simulink model "Modbus_Fixed_Breaker"  (Simulink 8.1)
settings: Solver=ode45  StartTime=0.0  StopTime=10.0  RelTol=1e-3
undefined symbols (not defined in the file or in its folder): Ts
libraries: powerlib x16, powerlib_extras x16, dspsigops x4, breakers_1ph_3ph x4, rtio_generic_modbus x4
settings Model: Creator=AI24004  LastModifiedBy=ed12083
settings DebuggingCC: FcnCallInpInsideContextMsg=EnableAllAsWarning

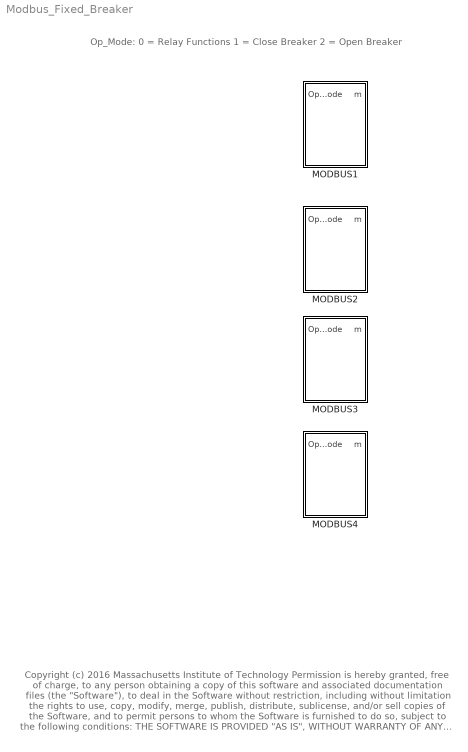
== system Modbus_Fixed_Breaker ==
  note: Op_Mode:
      | 0 = Relay Functions
      | 1 = Close Breaker
      | 2 = Open Breaker
  note: Copyright (c) 2016 Massachusetts Institute of Technology
      | Permission is hereby granted, free of charge, to any person obtaining a copy of this software and associated documentation files (the "Software"), to deal
      | in the Software without restriction, including without limitation the rights to use, copy, modify, merge, publish, distribute, sublicense, and/or sell copies of the
      | Software, and to permit persons to whom the Software is furnished to do so, subject to the following conditions:
      |
      | THE SOFTWARE IS PROVIDED "AS IS", WITHOUT WARRANTY OF ANY KIND, EXPRESS OR IMPLIED, INCLUDING BUT NOT LIMITED TO THE
      | WARRANTIES OF MERCHANTABILITY, FITNESS FOR A PARTICULAR PURPOSE AND NONINFRINGEMENT. IN NO EVENT SHALL THE AUTHORS
      | OR COPYRIGHT HOLDERS BE LIABLE FOR ANY CLAIM, DAMAGES OR OTHER LIABILITY, WHETHER IN AN ACTION OF CONTRACT, TORT OR
      | OTHERWISE, ARISING FROM, OUT OF OR IN CONNECTION WITH THE SOFTWARE OR THE USE OR OTHER DEALINGS IN THE SOFTWARE
  MODBUS1 : Subsystem  AncestorBlock=breakers_1ph_3ph/Protection  mask(Protection and Metering){IOC=15E3, TOC=1800, Ts=Ts, VRMSLL=13800, I_nom=200}
      mask prompts: IOC "IOC setting [A]"; TOC "TOC setting [A]"; Ts "Sampling Time [Sec]"; VRMSLL "Nominal Voltage [VRMSLL]"; I_nom "Continous Current [A]"
      mask help:
      | This block simulates the behavior of selected relay functions as well as metering equipment.
      | The block is intended to communicate with a microgrid controller providing it measurements, and switching controls.
      |
      | Supported relay functions (as of 06-15-2015):
      | 50/51: instantaneous and time-inverse overcurrent protection (moderate curve)
      mask Help:
      | This block simulates the behavior of selected relay functions as well as metering equipment (60 Hz - only).
      | The block is intended to communicate with a microgrid controller providing it measurements, and switching controls.
      | 
      | Supported relay functions (as of 06-15-2015):
      | 50/51: instantaneous and time-inverse overcurrent protection (moderate curve)
      | 
      | The input parameters are:
      | 0) Ts:  Sampling time [Seconds]
      | 1) State: 0 for relay logic mode, 1 to close the controlled breaker/switch,
      | and 2 to open the controlled breaker/switch
      | 2) TOC: Time-inverse overcurrent setting [Amperes]
      | 3) IOC: Instantaneous overcurrent setting [Amperes]
      | 
      | Metered parameters are:
      | 0) Status (0-closed, 1-open)
      | 1) Instantaneous voltage (abc)
      | 2) Instantaneous current (abc)
  MODBUS2 : Subsystem  AncestorBlock=breakers_1ph_3ph/Protection  mask(Protection and Metering){IOC=15E3, TOC=1800, Ts=Ts, VRMSLL=13800, I_nom=200}
      mask prompts: IOC "IOC setting [A]"; TOC "TOC setting [A]"; Ts "Sampling Time [Sec]"; VRMSLL "Nominal Voltage [VRMSLL]"; I_nom "Continous Current [A]"
      mask help:
      | This block simulates the behavior of selected relay functions as well as metering equipment.
      | The block is intended to communicate with a microgrid controller providing it measurements, and switching controls.
      |
      | Supported relay functions (as of 06-15-2015):
      | 50/51: instantaneous and time-inverse overcurrent protection (moderate curve)
      mask Help:
      | This block simulates the behavior of selected relay functions as well as metering equipment (60 Hz - only).
      | The block is intended to communicate with a microgrid controller providing it measurements, and switching controls.
      | 
      | Supported relay functions (as of 06-15-2015):
      | 50/51: instantaneous and time-inverse overcurrent protection (moderate curve)
      | 
      | The input parameters are:
      | 0) Ts:  Sampling time [Seconds]
      | 1) State: 0 for relay logic mode, 1 to close the controlled breaker/switch,
      | and 2 to open the controlled breaker/switch
      | 2) TOC: Time-inverse overcurrent setting [Amperes]
      | 3) IOC: Instantaneous overcurrent setting [Amperes]
      | 
      | Metered parameters are:
      | 0) Status (0-closed, 1-open)
      | 1) Instantaneous voltage (abc)
      | 2) Instantaneous current (abc)
  MODBUS3 : Subsystem  AncestorBlock=breakers_1ph_3ph/Protection  mask(Protection and Metering){IOC=15E3, TOC=1800, Ts=Ts, VRMSLL=13800, I_nom=200}
      mask prompts: IOC "IOC setting [A]"; TOC "TOC setting [A]"; Ts "Sampling Time [Sec]"; VRMSLL "Nominal Voltage [VRMSLL]"; I_nom "Continous Current [A]"
      mask help:
      | This block simulates the behavior of selected relay functions as well as metering equipment.
      | The block is intended to communicate with a microgrid controller providing it measurements, and switching controls.
      |
      | Supported relay functions (as of 06-15-2015):
      | 50/51: instantaneous and time-inverse overcurrent protection (moderate curve)
      mask Help:
      | This block simulates the behavior of selected relay functions as well as metering equipment (60 Hz - only).
      | The block is intended to communicate with a microgrid controller providing it measurements, and switching controls.
      | 
      | Supported relay functions (as of 06-15-2015):
      | 50/51: instantaneous and time-inverse overcurrent protection (moderate curve)
      | 
      | The input parameters are:
      | 0) Ts:  Sampling time [Seconds]
      | 1) State: 0 for relay logic mode, 1 to close the controlled breaker/switch,
      | and 2 to open the controlled breaker/switch
      | 2) TOC: Time-inverse overcurrent setting [Amperes]
      | 3) IOC: Instantaneous overcurrent setting [Amperes]
      | 
      | Metered parameters are:
      | 0) Status (0-closed, 1-open)
      | 1) Instantaneous voltage (abc)
      | 2) Instantaneous current (abc)
  MODBUS4 : Subsystem  AncestorBlock=breakers_1ph_3ph/Protection  mask(Protection and Metering){IOC=15E3, TOC=1800, Ts=Ts, VRMSLL=13800, I_nom=200}
      mask prompts: IOC "IOC setting [A]"; TOC "TOC setting [A]"; Ts "Sampling Time [Sec]"; VRMSLL "Nominal Voltage [VRMSLL]"; I_nom "Continous Current [A]"
      mask help:
      | This block simulates the behavior of selected relay functions as well as metering equipment.
      | The block is intended to communicate with a microgrid controller providing it measurements, and switching controls.
      |
      | Supported relay functions (as of 06-15-2015):
      | 50/51: instantaneous and time-inverse overcurrent protection (moderate curve)
      mask Help:
      | This block simulates the behavior of selected relay functions as well as metering equipment (60 Hz - only).
      | The block is intended to communicate with a microgrid controller providing it measurements, and switching controls.
      | 
      | Supported relay functions (as of 06-15-2015):
      | 50/51: instantaneous and time-inverse overcurrent protection (moderate curve)
      | 
      | The input parameters are:
      | 0) Ts:  Sampling time [Seconds]
      | 1) State: 0 for relay logic mode, 1 to close the controlled breaker/switch,
      | and 2 to open the controlled breaker/switch
      | 2) TOC: Time-inverse overcurrent setting [Amperes]
      | 3) IOC: Instantaneous overcurrent setting [Amperes]
      | 
      | Metered parameters are:
      | 0) Status (0-closed, 1-open)
      | 1) Instantaneous voltage (abc)
      | 2) Instantaneous current (abc)

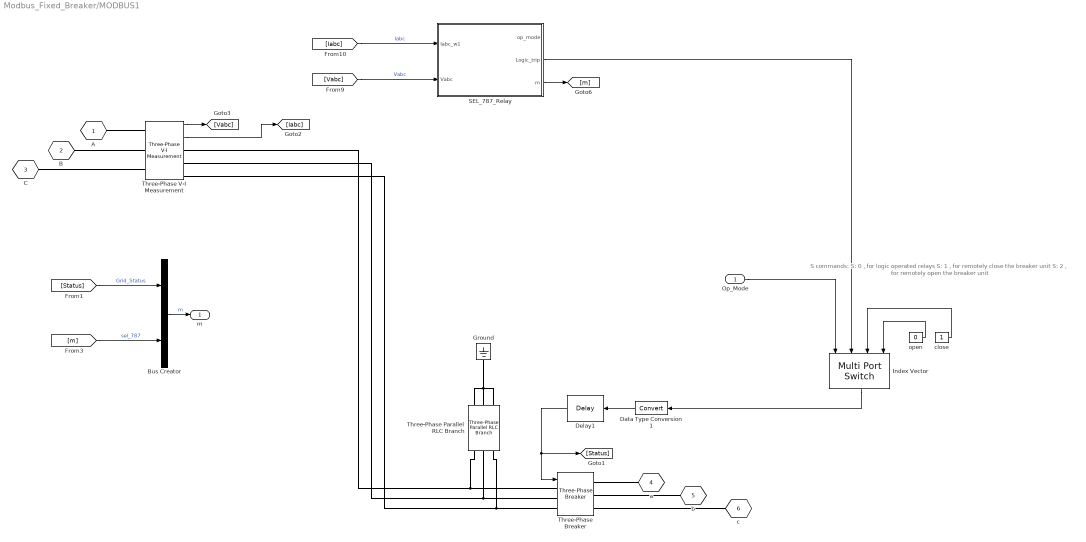
== system Modbus_Fixed_Breaker/MODBUS1 ==
  note: S commands:
      | S: 0 , for logic operated relays
      | S: 1 ,  for remotely close the breaker unit
      | S: 2 , for remotely open the breaker unit
  Op_Mode : Inport
  Bus Creator : BusCreator  Inputs=2
  Data Type Conversion1 : DataTypeConversion
  Delay1 : dspsigops/Delay  dly_unit=Samples  delay=lower((3/60)/Ts)  ic_detail=off  dif_ic_for_ch=off  dif_ic_for_dly=off  ic=1  reset_popup=None
  Ground : powerlib/Elements/Ground  LConnTagsString=a
  Index Vector : MultiPortSwitch  DataPortOrder=Zero-based contiguous  DataPortIndices={2,1,0}  zeroidx=on
  SEL_787_Relay : Subsystem
  Three-Phase Parallel RLC Branch : powerlib/Elements/Three-Phase Parallel RLC Branch  LConnTagsString=A|B|C  RConnTagsString=A|B|C  BranchType=RLC  Resistance=10e6  Inductance=1e-3  Capacitance=1e-6  Measurements=None
  Three-Phase V-I Measurement : powerlib/Measurements/Three-Phase V-I Measurement  VoltageMeasurement=phase-to-ground  SetLabelV=off  LabelV=Vabc  Vpu=off  VpuLL=off  CurrentMeasurement=yes  SetLabelI=off  LabelI=Iabc  Ipu=off  Pbase=100e6  Vbase=500e3  OutputType=Complex  PhasorSimulation=off  PSBequivalent=0
  Three-Phase Breaker : powerlib/Elements/Three-Phase Breaker  InitialState=closed  SwitchA=on  SwitchB=on  SwitchC=on  SwitchTimes="[1/60  5/60]"  External=on  BreakerResistance=1e-3  SnubberResistance=1e8  SnubberCapacitance=inf  Measurements=None
  close : Constant
  open : Constant  Value=0
  A : PMIOPort  Tag=PMCPort  Port=1  Side=Left
  B : PMIOPort  Tag=PMCPort  Port=2  Side=Left
  C : PMIOPort  Tag=PMCPort  Port=3  Side=Left
  a : PMIOPort  Tag=PMCPort  Port=4  Side=Right
  b : PMIOPort  Tag=PMCPort  Port=5  Side=Right
  c : PMIOPort  Tag=PMCPort  Port=6  Side=Right
  m : Outport
  wires:
  [m] -> Bus Creator/2  "sel_787"
  SEL_787_Relay/3(m) -> [m]
  Bus Creator/1 -> m/1  "m"
  [Status] -> Bus Creator/1  "Grid_Status"
  Delay1/1 -> [Status], Three-Phase Breaker/1
  Three-Phase V-I Measurement/1 -> [Vabc]
  Three-Phase V-I Measurement/2 -> [Iabc]
  open/1 -> Index Vector/4
  close/1 -> Index Vector/3
  Index Vector/1 -> Data Type Conversion1/1
  Data Type Conversion1/1 -> Delay1/1
  [Iabc] -> SEL_787_Relay/1(Iabc_w1)  "Iabc"
  [Vabc] -> SEL_787_Relay/2(Vabc)  "Vabc"
  SEL_787_Relay/2(Logic_trip) -> Index Vector/2
  Op_Mode/1 -> Index Vector/1
  connections:
  Three-Phase Parallel RLC Branch/RConn1 -- Three-Phase Breaker/LConn1 -- Three-Phase V-I Measurement/RConn1
  Three-Phase Parallel RLC Branch/RConn2 -- Three-Phase Breaker/LConn2 -- Three-Phase V-I Measurement/RConn2
  Three-Phase Parallel RLC Branch/RConn3 -- Three-Phase Breaker/LConn3 -- Three-Phase V-I Measurement/RConn3
  Three-Phase Breaker/RConn2 -- b/RConn1
  Three-Phase Breaker/RConn3 -- c/RConn1
  Three-Phase V-I Measurement/LConn1 -- A/RConn1
  a/RConn1 -- Three-Phase Breaker/RConn1
  C/RConn1 -- Three-Phase V-I Measurement/LConn3
  B/RConn1 -- Three-Phase V-I Measurement/LConn2
  Ground/LConn1 -- Three-Phase Parallel RLC Branch/LConn2 -- Three-Phase Parallel RLC Branch/LConn3 -- Three-Phase Parallel RLC Branch/LConn1

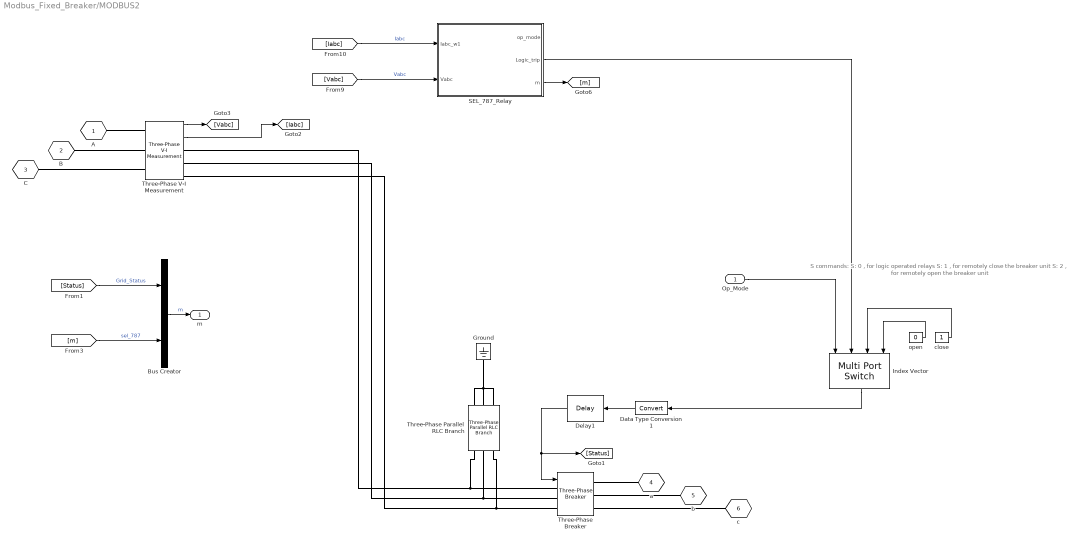
== system Modbus_Fixed_Breaker/MODBUS2 ==
  note: S commands:
      | S: 0 , for logic operated relays
      | S: 1 ,  for remotely close the breaker unit
      | S: 2 , for remotely open the breaker unit
  Op_Mode : Inport
  Bus Creator : BusCreator  Inputs=2
  Data Type Conversion1 : DataTypeConversion
  Delay1 : dspsigops/Delay  dly_unit=Samples  delay=lower((3/60)/Ts)  ic_detail=off  dif_ic_for_ch=off  dif_ic_for_dly=off  ic=1  reset_popup=None
  Ground : powerlib/Elements/Ground  LConnTagsString=a
  Index Vector : MultiPortSwitch  DataPortOrder=Zero-based contiguous  DataPortIndices={2,1,0}  zeroidx=on
  SEL_787_Relay : Subsystem
  Three-Phase Parallel RLC Branch : powerlib/Elements/Three-Phase Parallel RLC Branch  LConnTagsString=A|B|C  RConnTagsString=A|B|C  BranchType=RLC  Resistance=10e6  Inductance=1e-3  Capacitance=1e-6  Measurements=None
  Three-Phase V-I Measurement : powerlib/Measurements/Three-Phase V-I Measurement  VoltageMeasurement=phase-to-ground  SetLabelV=off  LabelV=Vabc  Vpu=off  VpuLL=off  CurrentMeasurement=yes  SetLabelI=off  LabelI=Iabc  Ipu=off  Pbase=100e6  Vbase=500e3  OutputType=Complex  PhasorSimulation=off  PSBequivalent=0
  Three-Phase Breaker : powerlib/Elements/Three-Phase Breaker  InitialState=closed  SwitchA=on  SwitchB=on  SwitchC=on  SwitchTimes="[1/60  5/60]"  External=on  BreakerResistance=1e-3  SnubberResistance=1e8  SnubberCapacitance=inf  Measurements=None
  close : Constant
  open : Constant  Value=0
  A : PMIOPort  Tag=PMCPort  Port=1  Side=Left
  B : PMIOPort  Tag=PMCPort  Port=2  Side=Left
  C : PMIOPort  Tag=PMCPort  Port=3  Side=Left
  a : PMIOPort  Tag=PMCPort  Port=4  Side=Right
  b : PMIOPort  Tag=PMCPort  Port=5  Side=Right
  c : PMIOPort  Tag=PMCPort  Port=6  Side=Right
  m : Outport
  wires:
  [m] -> Bus Creator/2  "sel_787"
  SEL_787_Relay/3(m) -> [m]
  Bus Creator/1 -> m/1  "m"
  [Status] -> Bus Creator/1  "Grid_Status"
  Delay1/1 -> [Status], Three-Phase Breaker/1
  Three-Phase V-I Measurement/1 -> [Vabc]
  Three-Phase V-I Measurement/2 -> [Iabc]
  open/1 -> Index Vector/4
  close/1 -> Index Vector/3
  Index Vector/1 -> Data Type Conversion1/1
  Data Type Conversion1/1 -> Delay1/1
  [Iabc] -> SEL_787_Relay/1(Iabc_w1)  "Iabc"
  [Vabc] -> SEL_787_Relay/2(Vabc)  "Vabc"
  SEL_787_Relay/2(Logic_trip) -> Index Vector/2
  Op_Mode/1 -> Index Vector/1
  connections:
  Three-Phase V-I Measurement/RConn1 -- Three-Phase Parallel RLC Branch/RConn1 -- Three-Phase Breaker/LConn1
  Three-Phase V-I Measurement/RConn2 -- Three-Phase Parallel RLC Branch/RConn2 -- Three-Phase Breaker/LConn2
  Three-Phase V-I Measurement/RConn3 -- Three-Phase Parallel RLC Branch/RConn3 -- Three-Phase Breaker/LConn3
  Three-Phase Breaker/RConn2 -- b/RConn1
  Three-Phase Breaker/RConn3 -- c/RConn1
  Three-Phase V-I Measurement/LConn1 -- A/RConn1
  a/RConn1 -- Three-Phase Breaker/RConn1
  C/RConn1 -- Three-Phase V-I Measurement/LConn3
  B/RConn1 -- Three-Phase V-I Measurement/LConn2
  Ground/LConn1 -- Three-Phase Parallel RLC Branch/LConn2 -- Three-Phase Parallel RLC Branch/LConn3 -- Three-Phase Parallel RLC Branch/LConn1

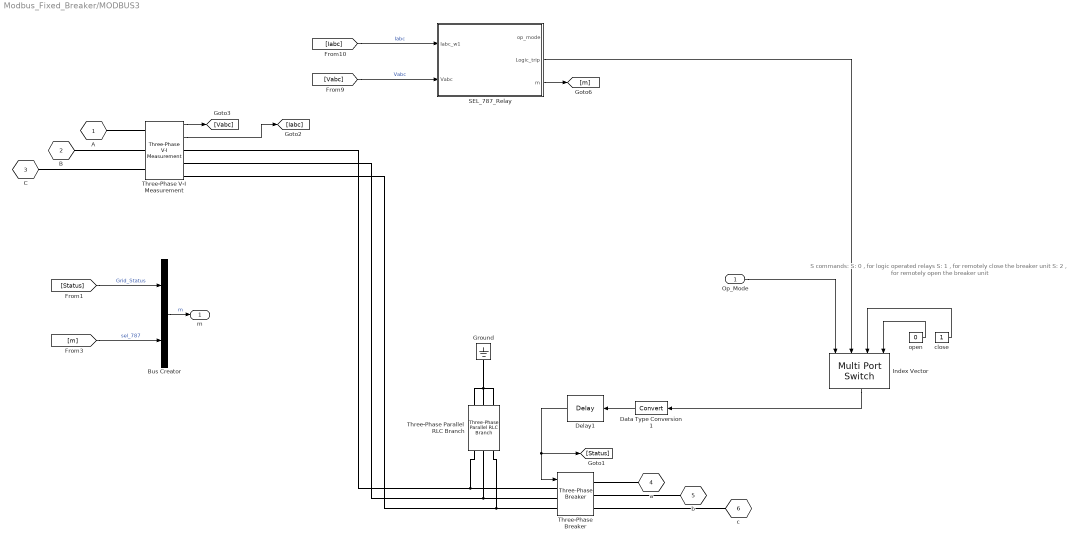
== system Modbus_Fixed_Breaker/MODBUS3 ==
  note: S commands:
      | S: 0 , for logic operated relays
      | S: 1 ,  for remotely close the breaker unit
      | S: 2 , for remotely open the breaker unit
  Op_Mode : Inport
  Bus Creator : BusCreator  Inputs=2
  Data Type Conversion1 : DataTypeConversion
  Delay1 : dspsigops/Delay  dly_unit=Samples  delay=lower((3/60)/Ts)  ic_detail=off  dif_ic_for_ch=off  dif_ic_for_dly=off  ic=1  reset_popup=None
  Ground : powerlib/Elements/Ground  LConnTagsString=a
  Index Vector : MultiPortSwitch  DataPortOrder=Zero-based contiguous  DataPortIndices={2,1,0}  zeroidx=on
  SEL_787_Relay : Subsystem
  Three-Phase Parallel RLC Branch : powerlib/Elements/Three-Phase Parallel RLC Branch  LConnTagsString=A|B|C  RConnTagsString=A|B|C  BranchType=RLC  Resistance=10e6  Inductance=1e-3  Capacitance=1e-6  Measurements=None
  Three-Phase V-I Measurement : powerlib/Measurements/Three-Phase V-I Measurement  VoltageMeasurement=phase-to-ground  SetLabelV=off  LabelV=Vabc  Vpu=off  VpuLL=off  CurrentMeasurement=yes  SetLabelI=off  LabelI=Iabc  Ipu=off  Pbase=100e6  Vbase=500e3  OutputType=Complex  PhasorSimulation=off  PSBequivalent=0
  Three-Phase Breaker : powerlib/Elements/Three-Phase Breaker  InitialState=closed  SwitchA=on  SwitchB=on  SwitchC=on  SwitchTimes="[1/60  5/60]"  External=on  BreakerResistance=1e-3  SnubberResistance=1e8  SnubberCapacitance=inf  Measurements=None
  close : Constant
  open : Constant  Value=0
  A : PMIOPort  Tag=PMCPort  Port=1  Side=Left
  B : PMIOPort  Tag=PMCPort  Port=2  Side=Left
  C : PMIOPort  Tag=PMCPort  Port=3  Side=Left
  a : PMIOPort  Tag=PMCPort  Port=4  Side=Right
  b : PMIOPort  Tag=PMCPort  Port=5  Side=Right
  c : PMIOPort  Tag=PMCPort  Port=6  Side=Right
  m : Outport
  wires:
  [m] -> Bus Creator/2  "sel_787"
  SEL_787_Relay/3(m) -> [m]
  Bus Creator/1 -> m/1  "m"
  [Status] -> Bus Creator/1  "Grid_Status"
  Delay1/1 -> [Status], Three-Phase Breaker/1
  Three-Phase V-I Measurement/1 -> [Vabc]
  Three-Phase V-I Measurement/2 -> [Iabc]
  open/1 -> Index Vector/4
  close/1 -> Index Vector/3
  Index Vector/1 -> Data Type Conversion1/1
  Data Type Conversion1/1 -> Delay1/1
  [Iabc] -> SEL_787_Relay/1(Iabc_w1)  "Iabc"
  [Vabc] -> SEL_787_Relay/2(Vabc)  "Vabc"
  SEL_787_Relay/2(Logic_trip) -> Index Vector/2
  Op_Mode/1 -> Index Vector/1
  connections:
  Three-Phase V-I Measurement/RConn1 -- Three-Phase Parallel RLC Branch/RConn1 -- Three-Phase Breaker/LConn1
  Three-Phase V-I Measurement/RConn2 -- Three-Phase Parallel RLC Branch/RConn2 -- Three-Phase Breaker/LConn2
  Three-Phase V-I Measurement/RConn3 -- Three-Phase Parallel RLC Branch/RConn3 -- Three-Phase Breaker/LConn3
  Three-Phase Breaker/RConn2 -- b/RConn1
  Three-Phase Breaker/RConn3 -- c/RConn1
  Three-Phase V-I Measurement/LConn1 -- A/RConn1
  a/RConn1 -- Three-Phase Breaker/RConn1
  C/RConn1 -- Three-Phase V-I Measurement/LConn3
  B/RConn1 -- Three-Phase V-I Measurement/LConn2
  Ground/LConn1 -- Three-Phase Parallel RLC Branch/LConn2 -- Three-Phase Parallel RLC Branch/LConn3 -- Three-Phase Parallel RLC Branch/LConn1

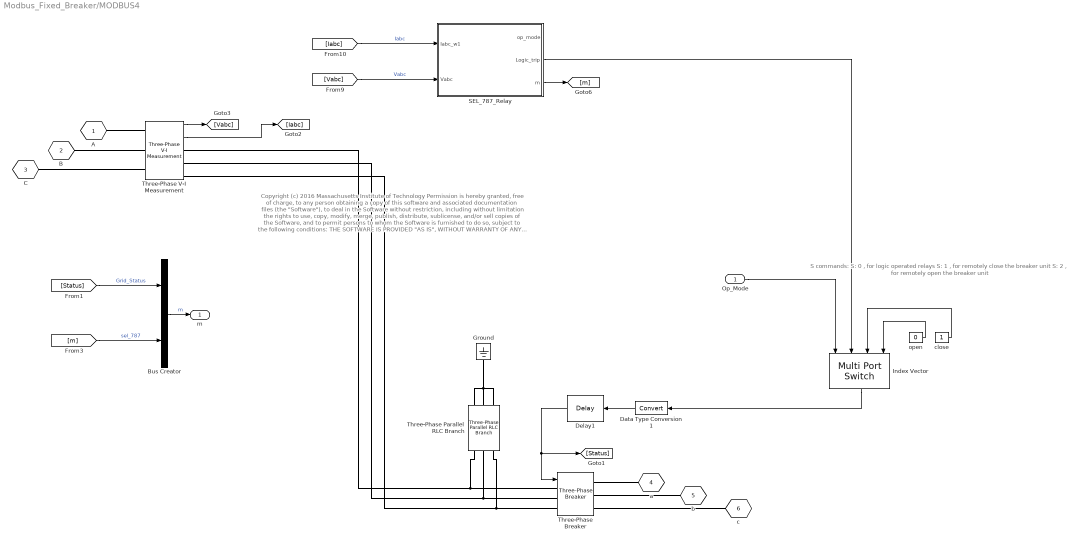
== system Modbus_Fixed_Breaker/MODBUS4 ==
  note: S commands:
      | S: 0 , for logic operated relays
      | S: 1 ,  for remotely close the breaker unit
      | S: 2 , for remotely open the breaker unit
  note: Copyright (c) 2016 Massachusetts Institute of Technology
      | Permission is hereby granted, free of charge, to any person obtaining a copy of this software and associated documentation files (the "Software"), to deal
      | in the Software without restriction, including without limitation the rights to use, copy, modify, merge, publish, distribute, sublicense, and/or sell copies of the
      | Software, and to permit persons to whom the Software is furnished to do so, subject to the following conditions:
      |
      | THE SOFTWARE IS PROVIDED "AS IS", WITHOUT WARRANTY OF ANY KIND, EXPRESS OR IMPLIED, INCLUDING BUT NOT LIMITED TO THE
      | WARRANTIES OF MERCHANTABILITY, FITNESS FOR A PARTICULAR PURPOSE AND NONINFRINGEMENT. IN NO EVENT SHALL THE AUTHORS
      | OR COPYRIGHT HOLDERS BE LIABLE FOR ANY CLAIM, DAMAGES OR OTHER LIABILITY, WHETHER IN AN ACTION OF CONTRACT, TORT OR
      | OTHERWISE, ARISING FROM, OUT OF OR IN CONNECTION WITH THE SOFTWARE OR THE USE OR OTHER DEALINGS IN THE SOFTWARE
  Op_Mode : Inport
  Bus Creator : BusCreator  Inputs=2
  Data Type Conversion1 : DataTypeConversion
  Delay1 : dspsigops/Delay  dly_unit=Samples  delay=lower((3/60)/Ts)  ic_detail=off  dif_ic_for_ch=off  dif_ic_for_dly=off  ic=1  reset_popup=None
  Ground : powerlib/Elements/Ground  LConnTagsString=a
  Index Vector : MultiPortSwitch  DataPortOrder=Zero-based contiguous  DataPortIndices={2,1,0}  zeroidx=on
  SEL_787_Relay : Subsystem
  Three-Phase Parallel RLC Branch : powerlib/Elements/Three-Phase Parallel RLC Branch  LConnTagsString=A|B|C  RConnTagsString=A|B|C  BranchType=RLC  Resistance=10e6  Inductance=1e-3  Capacitance=1e-6  Measurements=None
  Three-Phase V-I Measurement : powerlib/Measurements/Three-Phase V-I Measurement  VoltageMeasurement=phase-to-ground  SetLabelV=off  LabelV=Vabc  Vpu=off  VpuLL=off  CurrentMeasurement=yes  SetLabelI=off  LabelI=Iabc  Ipu=off  Pbase=100e6  Vbase=500e3  OutputType=Complex  PhasorSimulation=off  PSBequivalent=0
  Three-Phase Breaker : powerlib/Elements/Three-Phase Breaker  InitialState=closed  SwitchA=on  SwitchB=on  SwitchC=on  SwitchTimes="[1/60  5/60]"  External=on  BreakerResistance=1e-3  SnubberResistance=1e8  SnubberCapacitance=inf  Measurements=None
  close : Constant
  open : Constant  Value=0
  A : PMIOPort  Tag=PMCPort  Port=1  Side=Left
  B : PMIOPort  Tag=PMCPort  Port=2  Side=Left
  C : PMIOPort  Tag=PMCPort  Port=3  Side=Left
  a : PMIOPort  Tag=PMCPort  Port=4  Side=Right
  b : PMIOPort  Tag=PMCPort  Port=5  Side=Right
  c : PMIOPort  Tag=PMCPort  Port=6  Side=Right
  m : Outport
  wires:
  [m] -> Bus Creator/2  "sel_787"
  SEL_787_Relay/3(m) -> [m]
  Bus Creator/1 -> m/1  "m"
  [Status] -> Bus Creator/1  "Grid_Status"
  Delay1/1 -> [Status], Three-Phase Breaker/1
  Three-Phase V-I Measurement/1 -> [Vabc]
  Three-Phase V-I Measurement/2 -> [Iabc]
  open/1 -> Index Vector/4
  close/1 -> Index Vector/3
  Index Vector/1 -> Data Type Conversion1/1
  Data Type Conversion1/1 -> Delay1/1
  [Iabc] -> SEL_787_Relay/1(Iabc_w1)  "Iabc"
  [Vabc] -> SEL_787_Relay/2(Vabc)  "Vabc"
  SEL_787_Relay/2(Logic_trip) -> Index Vector/2
  Op_Mode/1 -> Index Vector/1
  connections:
  Three-Phase V-I Measurement/RConn1 -- Three-Phase Parallel RLC Branch/RConn1 -- Three-Phase Breaker/LConn1
  Three-Phase V-I Measurement/RConn2 -- Three-Phase Parallel RLC Branch/RConn2 -- Three-Phase Breaker/LConn2
  Three-Phase V-I Measurement/RConn3 -- Three-Phase Parallel RLC Branch/RConn3 -- Three-Phase Breaker/LConn3
  Three-Phase Breaker/RConn2 -- b/RConn1
  Three-Phase Breaker/RConn3 -- c/RConn1
  Three-Phase V-I Measurement/LConn1 -- A/RConn1
  a/RConn1 -- Three-Phase Breaker/RConn1
  C/RConn1 -- Three-Phase V-I Measurement/LConn3
  B/RConn1 -- Three-Phase V-I Measurement/LConn2
  Ground/LConn1 -- Three-Phase Parallel RLC Branch/LConn2 -- Three-Phase Parallel RLC Branch/LConn3 -- Three-Phase Parallel RLC Branch/LConn1

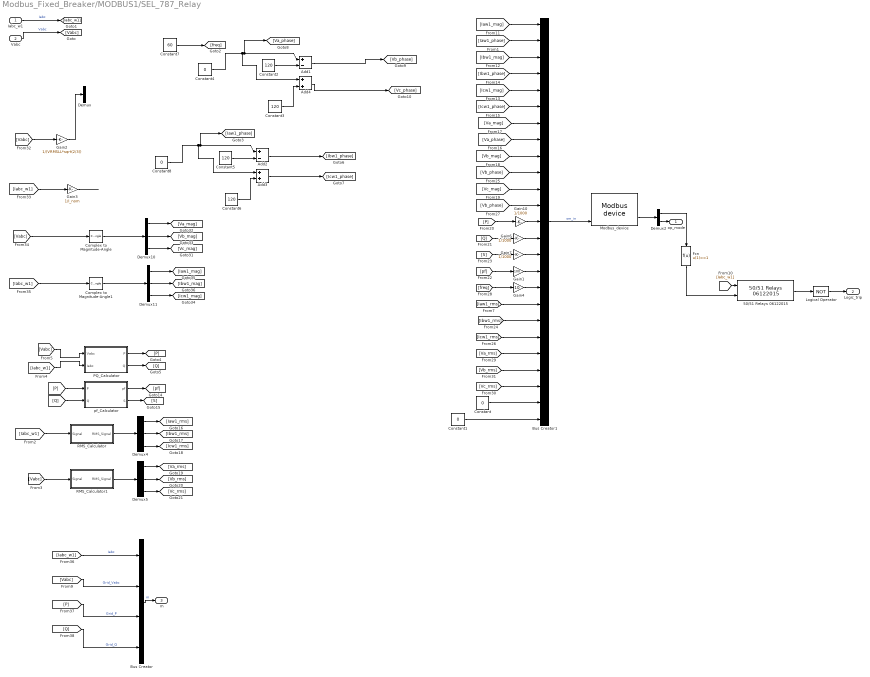
== system Modbus_Fixed_Breaker/MODBUS1/SEL_787_Relay ==
  Iabc_w1 : Inport
  Vabc : Inport  Port=2
  50/51 Relays 06122015 : breakers_1ph_3ph/50//51 Relays 06122015  TOC=TOC  IOC=IOC  Ts=Ts
  Add1 : Sum  Inputs=+-
  Add2 : Sum  Inputs=+-
  Add3 : Sum
  Add4 : Sum
  Bus Creator : BusCreator
  Bus Creator1 : BusCreator  Inputs=25
  Complex to Magnitude-Angle : ComplexToMagnitudeAngle  Output=Magnitude
  Complex to Magnitude-Angle1 : ComplexToMagnitudeAngle  Output=Magnitude
  Constant{,1,4,8} (4 alike) : Constant  Value=0
  Constant{2..3,5..6} (4 alike) : Constant  Value=120
  Constant7 : Constant  Value=60
  Demux{,4..5,10..11} (5 alike) : Demux  Outputs=3
  Demux2 : Demux  Outputs=2
  Fcn : Fcn  Expr=u(1)==1
  Gain1 : Gain  Gain=100
  Gain10 : Gain  Gain=1/1000
  Gain2 : Gain  Gain=1/(VRMSLL*sqrt(2/3))
  Gain3 : Gain  Gain=1/I_nom
  Gain4 : Gain  Gain=10
  Gain6 : Gain  Gain=1/1000
  Gain7 : Gain  Gain=1/1000
  Logical Operator : Logic  Operator=NOT  AllPortsSameDT=off  OutDataTypeStr=boolean
  Modbus_device : rtio_generic_modbus/Modbus device  conf_name=relay_slave_cfg1.opal  conf_name_mask=relay_slave_cfg1.xls  sample_time=Ts
  PQ_Calculator : Subsystem
  RMS_Calculator : Subsystem
  RMS_Calculator1 : Subsystem
  pf_Calculator : Subsystem
  op_mode : Outport
  Logic_trip : Outport  Port=2
  m : Outport  Port=3
  wires:
  Gain4/1 -> Bus Creator1/17
  Gain1/1 -> Bus Creator1/16
  [pf] -> Gain1/1
  [freq] -> Gain4/1
  Constant4/1 -> Add4/1, [Va_phase], Add1/1
  Add4/1 -> [Vc_phase]
  Add1/1 -> [Vb_phase]
  Constant3/1 -> Add4/2
  Constant2/1 -> Add1/2
  Constant8/1 -> Add3/1, [Iaw1_phase], Add2/1
  Add3/1 -> [Icw1_phase]
  Add2/1 -> [Ibw1_phase]
  Constant6/1 -> Add3/2
  Constant5/1 -> Add2/2
  Constant7/1 -> [freq]
  pf_Calculator/2(S) -> [S]
  Bus Creator1/1 -> Modbus_device/4  "sm_in"
  Modbus_device/2 -> Demux2/1
  [Q] -> Bus Creator/4  "Grid_Q"
  [P] -> Bus Creator/3  "Grid_P"
  [Vabc] -> Bus Creator/2  "Grid_Vabc"
  [Iabc_w1] -> Bus Creator/1  "Iabc"
  Bus Creator/1 -> m/1  "m"
  Iabc_w1/1 -> [Iabc_w1]  "Iabc"
  Vabc/1 -> [Vabc]  "Vabc"
  [Vabc] -> PQ_Calculator/1(Vabc)
  [Iabc_w1] -> PQ_Calculator/2(Iabc)
  [Iaw1_mag] -> Bus Creator1/1
  [P] -> Gain10/1
  [Q] -> Gain6/1
  [S] -> Gain7/1
  pf_Calculator/1(pf) -> [pf]
  [P] -> pf_Calculator/1(P)
  [Q] -> pf_Calculator/2(Q)
  PQ_Calculator/1(P) -> [P]
  PQ_Calculator/2(Q) -> [Q]
  [Iabc_w1] -> RMS_Calculator/1(Signal)
  [Vabc] -> RMS_Calculator1/1(Signal)
  RMS_Calculator/1(RMS_Signal) -> Demux4/1
  RMS_Calculator1/1(RMS_Signal) -> Demux5/1
  Demux4/3 -> [Icw1_rms]
  Demux4/2 -> [Ibw1_rms]
  Demux4/1 -> [Iaw1_rms]
  Demux5/1 -> [Va_rms]
  Demux5/2 -> [Vb_rms]
  Demux5/3 -> [Vc_rms]
  Demux2/1 -> Fcn/1
  Fcn/1 -> 50/51 Relays 06122015/2
  [Iabc_w1] -> 50/51 Relays 06122015/1
  50/51 Relays 06122015/1 -> Logical Operator/1
  [Ibw1_mag] -> Bus Creator1/3
  [Icw1_mag] -> Bus Creator1/5
  [Va_mag] -> Bus Creator1/7
  [Vb_mag] -> Bus Creator1/9
  [Vc_mag] -> Bus Creator1/11
  Gain10/1 -> Bus Creator1/13
  Gain6/1 -> Bus Creator1/14
  Gain7/1 -> Bus Creator1/15
  [Iaw1_rms] -> Bus Creator1/18
  [Icw1_rms] -> Bus Creator1/20
  [Ibw1_rms] -> Bus Creator1/19
  [Va_rms] -> Bus Creator1/21
  [Vb_rms] -> Bus Creator1/22
  [Vc_rms] -> Bus Creator1/23
  Logical Operator/1 -> Logic_trip/1
  Demux2/2 -> op_mode/1
  [Iaw1_phase] -> Bus Creator1/2
  [Ibw1_phase] -> Bus Creator1/4
  [Icw1_phase] -> Bus Creator1/6
  [Va_phase] -> Bus Creator1/8
  [Vb_phase] -> Bus Creator1/10
  [Vb_phase] -> Bus Creator1/12
  Constant/1 -> Bus Creator1/24
  Constant1/1 -> Bus Creator1/25
  [Vabc] -> Gain2/1
  Gain2/1 -> Demux/1
  [Iabc_w1] -> Gain3/1
  Gain3/1 -> ?
  Demux10/1 -> [Va_mag]
  Demux10/2 -> [Vb_mag]
  Demux10/3 -> [Vc_mag]
  Complex to Magnitude-Angle/1 -> Demux10/1
  [Vabc] -> Complex to Magnitude-Angle/1
  Complex to Magnitude-Angle1/1 -> Demux11/1
  [Iabc_w1] -> Complex to Magnitude-Angle1/1
  Demux11/1 -> [Iaw1_mag]
  Demux11/2 -> [Ibw1_mag]
  Demux11/3 -> [Icw1_mag]

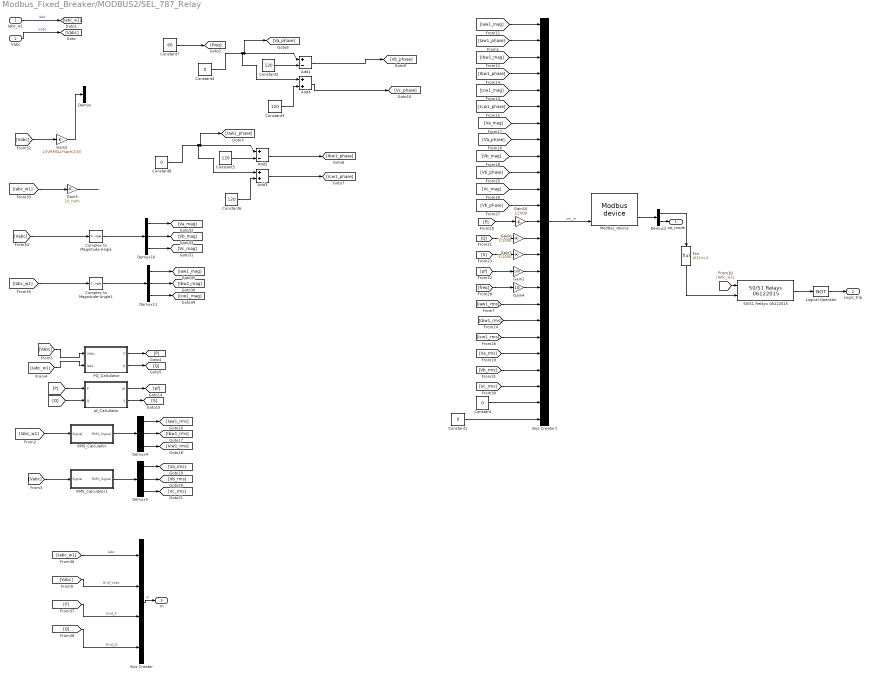
== system Modbus_Fixed_Breaker/MODBUS2/SEL_787_Relay ==
  Iabc_w1 : Inport
  Vabc : Inport  Port=2
  50/51 Relays 06122015 : breakers_1ph_3ph/50//51 Relays 06122015  TOC=TOC  IOC=IOC  Ts=Ts
  Add1 : Sum  Inputs=+-
  Add2 : Sum  Inputs=+-
  Add3 : Sum
  Add4 : Sum
  Bus Creator : BusCreator
  Bus Creator1 : BusCreator  Inputs=25
  Complex to Magnitude-Angle : ComplexToMagnitudeAngle  Output=Magnitude
  Complex to Magnitude-Angle1 : ComplexToMagnitudeAngle  Output=Magnitude
  Constant{,1,4,8} (4 alike) : Constant  Value=0
  Constant{2..3,5..6} (4 alike) : Constant  Value=120
  Constant7 : Constant  Value=60
  Demux{,4..5,10..11} (5 alike) : Demux  Outputs=3
  Demux2 : Demux  Outputs=2
  Fcn : Fcn  Expr=u(1)==1
  Gain1 : Gain  Gain=100
  Gain10 : Gain  Gain=1/1000
  Gain2 : Gain  Gain=1/(VRMSLL*sqrt(2/3))
  Gain3 : Gain  Gain=1/I_nom
  Gain4 : Gain  Gain=10
  Gain6 : Gain  Gain=1/1000
  Gain7 : Gain  Gain=1/1000
  Logical Operator : Logic  Operator=NOT  AllPortsSameDT=off  OutDataTypeStr=boolean
  Modbus_device : rtio_generic_modbus/Modbus device  conf_name=relay_slave_cfg1.opal  conf_name_mask=relay_slave_cfg2.xls  sample_time=Ts
  PQ_Calculator : Subsystem
  RMS_Calculator : Subsystem
  RMS_Calculator1 : Subsystem
  pf_Calculator : Subsystem
  op_mode : Outport
  Logic_trip : Outport  Port=2
  m : Outport  Port=3
  wires:
  Gain4/1 -> Bus Creator1/17
  Gain1/1 -> Bus Creator1/16
  [pf] -> Gain1/1
  [freq] -> Gain4/1
  Constant4/1 -> Add4/1, [Va_phase], Add1/1
  Add4/1 -> [Vc_phase]
  Add1/1 -> [Vb_phase]
  Constant3/1 -> Add4/2
  Constant2/1 -> Add1/2
  Constant8/1 -> Add3/1, [Iaw1_phase], Add2/1
  Add3/1 -> [Icw1_phase]
  Add2/1 -> [Ibw1_phase]
  Constant6/1 -> Add3/2
  Constant5/1 -> Add2/2
  Constant7/1 -> [freq]
  pf_Calculator/2(S) -> [S]
  Bus Creator1/1 -> Modbus_device/4  "sm_in"
  Modbus_device/2 -> Demux2/1
  [Q] -> Bus Creator/4  "Grid_Q"
  [P] -> Bus Creator/3  "Grid_P"
  [Vabc] -> Bus Creator/2  "Grid_Vabc"
  [Iabc_w1] -> Bus Creator/1  "Iabc"
  Bus Creator/1 -> m/1  "m"
  Iabc_w1/1 -> [Iabc_w1]  "Iabc"
  Vabc/1 -> [Vabc]  "Vabc"
  [Vabc] -> PQ_Calculator/1(Vabc)
  [Iabc_w1] -> PQ_Calculator/2(Iabc)
  [Iaw1_mag] -> Bus Creator1/1
  [P] -> Gain10/1
  [Q] -> Gain6/1
  [S] -> Gain7/1
  pf_Calculator/1(pf) -> [pf]
  [P] -> pf_Calculator/1(P)
  [Q] -> pf_Calculator/2(Q)
  PQ_Calculator/1(P) -> [P]
  PQ_Calculator/2(Q) -> [Q]
  [Iabc_w1] -> RMS_Calculator/1(Signal)
  [Vabc] -> RMS_Calculator1/1(Signal)
  RMS_Calculator/1(RMS_Signal) -> Demux4/1
  RMS_Calculator1/1(RMS_Signal) -> Demux5/1
  Demux4/3 -> [Icw1_rms]
  Demux4/2 -> [Ibw1_rms]
  Demux4/1 -> [Iaw1_rms]
  Demux5/1 -> [Va_rms]
  Demux5/2 -> [Vb_rms]
  Demux5/3 -> [Vc_rms]
  Demux2/1 -> Fcn/1
  Fcn/1 -> 50/51 Relays 06122015/2
  [Iabc_w1] -> 50/51 Relays 06122015/1
  50/51 Relays 06122015/1 -> Logical Operator/1
  [Ibw1_mag] -> Bus Creator1/3
  [Icw1_mag] -> Bus Creator1/5
  [Va_mag] -> Bus Creator1/7
  [Vb_mag] -> Bus Creator1/9
  [Vc_mag] -> Bus Creator1/11
  Gain10/1 -> Bus Creator1/13
  Gain6/1 -> Bus Creator1/14
  Gain7/1 -> Bus Creator1/15
  [Iaw1_rms] -> Bus Creator1/18
  [Icw1_rms] -> Bus Creator1/20
  [Ibw1_rms] -> Bus Creator1/19
  [Va_rms] -> Bus Creator1/21
  [Vb_rms] -> Bus Creator1/22
  [Vc_rms] -> Bus Creator1/23
  Logical Operator/1 -> Logic_trip/1
  Demux2/2 -> op_mode/1
  [Iaw1_phase] -> Bus Creator1/2
  [Ibw1_phase] -> Bus Creator1/4
  [Icw1_phase] -> Bus Creator1/6
  [Va_phase] -> Bus Creator1/8
  [Vb_phase] -> Bus Creator1/10
  [Vb_phase] -> Bus Creator1/12
  Constant/1 -> Bus Creator1/24
  Constant1/1 -> Bus Creator1/25
  [Vabc] -> Gain2/1
  Gain2/1 -> Demux/1
  [Iabc_w1] -> Gain3/1
  Gain3/1 -> ?
  Demux10/1 -> [Va_mag]
  Demux10/2 -> [Vb_mag]
  Demux10/3 -> [Vc_mag]
  Complex to Magnitude-Angle/1 -> Demux10/1
  [Vabc] -> Complex to Magnitude-Angle/1
  Complex to Magnitude-Angle1/1 -> Demux11/1
  [Iabc_w1] -> Complex to Magnitude-Angle1/1
  Demux11/1 -> [Iaw1_mag]
  Demux11/2 -> [Ibw1_mag]
  Demux11/3 -> [Icw1_mag]

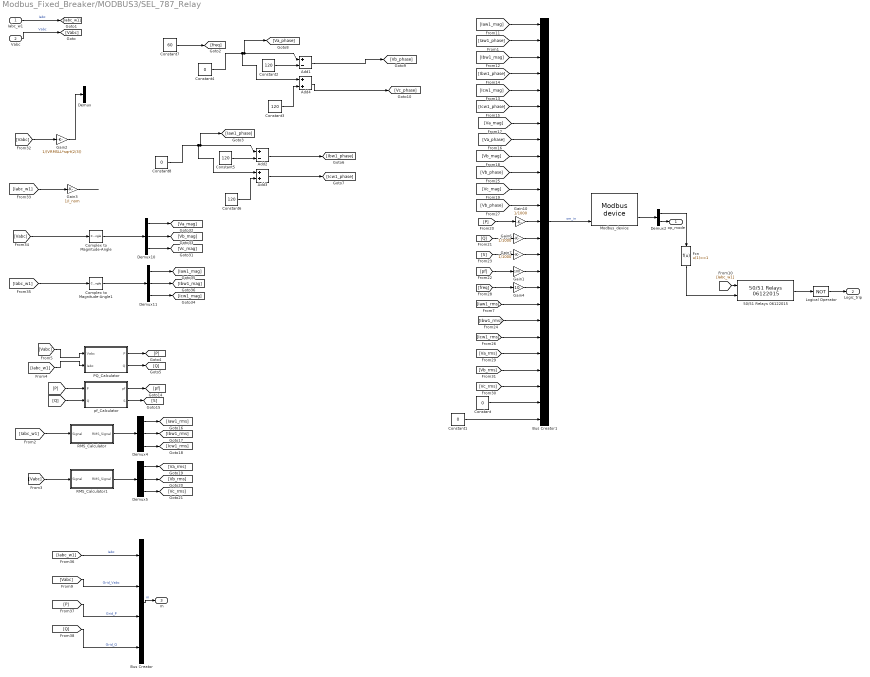
== system Modbus_Fixed_Breaker/MODBUS3/SEL_787_Relay ==
  Iabc_w1 : Inport
  Vabc : Inport  Port=2
  50/51 Relays 06122015 : breakers_1ph_3ph/50//51 Relays 06122015  TOC=TOC  IOC=IOC  Ts=Ts
  Add1 : Sum  Inputs=+-
  Add2 : Sum  Inputs=+-
  Add3 : Sum
  Add4 : Sum
  Bus Creator : BusCreator
  Bus Creator1 : BusCreator  Inputs=25
  Complex to Magnitude-Angle : ComplexToMagnitudeAngle  Output=Magnitude
  Complex to Magnitude-Angle1 : ComplexToMagnitudeAngle  Output=Magnitude
  Constant{,1,4,8} (4 alike) : Constant  Value=0
  Constant{2..3,5..6} (4 alike) : Constant  Value=120
  Constant7 : Constant  Value=60
  Demux{,4..5,10..11} (5 alike) : Demux  Outputs=3
  Demux2 : Demux  Outputs=2
  Fcn : Fcn  Expr=u(1)==1
  Gain1 : Gain  Gain=100
  Gain10 : Gain  Gain=1/1000
  Gain2 : Gain  Gain=1/(VRMSLL*sqrt(2/3))
  Gain3 : Gain  Gain=1/I_nom
  Gain4 : Gain  Gain=10
  Gain6 : Gain  Gain=1/1000
  Gain7 : Gain  Gain=1/1000
  Logical Operator : Logic  Operator=NOT  AllPortsSameDT=off  OutDataTypeStr=boolean
  Modbus_device : rtio_generic_modbus/Modbus device  conf_name=relay_slave_cfg1.opal  conf_name_mask=relay_slave_cfg3.xls  sample_time=Ts
  PQ_Calculator : Subsystem
  RMS_Calculator : Subsystem
  RMS_Calculator1 : Subsystem
  pf_Calculator : Subsystem
  op_mode : Outport
  Logic_trip : Outport  Port=2
  m : Outport  Port=3
  wires:
  Gain4/1 -> Bus Creator1/17
  Gain1/1 -> Bus Creator1/16
  [pf] -> Gain1/1
  [freq] -> Gain4/1
  Constant4/1 -> Add4/1, [Va_phase], Add1/1
  Add4/1 -> [Vc_phase]
  Add1/1 -> [Vb_phase]
  Constant3/1 -> Add4/2
  Constant2/1 -> Add1/2
  Constant8/1 -> Add3/1, [Iaw1_phase], Add2/1
  Add3/1 -> [Icw1_phase]
  Add2/1 -> [Ibw1_phase]
  Constant6/1 -> Add3/2
  Constant5/1 -> Add2/2
  Constant7/1 -> [freq]
  pf_Calculator/2(S) -> [S]
  Bus Creator1/1 -> Modbus_device/4  "sm_in"
  Modbus_device/2 -> Demux2/1
  [Q] -> Bus Creator/4  "Grid_Q"
  [P] -> Bus Creator/3  "Grid_P"
  [Vabc] -> Bus Creator/2  "Grid_Vabc"
  [Iabc_w1] -> Bus Creator/1  "Iabc"
  Bus Creator/1 -> m/1  "m"
  Iabc_w1/1 -> [Iabc_w1]  "Iabc"
  Vabc/1 -> [Vabc]  "Vabc"
  [Vabc] -> PQ_Calculator/1(Vabc)
  [Iabc_w1] -> PQ_Calculator/2(Iabc)
  [Iaw1_mag] -> Bus Creator1/1
  [P] -> Gain10/1
  [Q] -> Gain6/1
  [S] -> Gain7/1
  pf_Calculator/1(pf) -> [pf]
  [P] -> pf_Calculator/1(P)
  [Q] -> pf_Calculator/2(Q)
  PQ_Calculator/1(P) -> [P]
  PQ_Calculator/2(Q) -> [Q]
  [Iabc_w1] -> RMS_Calculator/1(Signal)
  [Vabc] -> RMS_Calculator1/1(Signal)
  RMS_Calculator/1(RMS_Signal) -> Demux4/1
  RMS_Calculator1/1(RMS_Signal) -> Demux5/1
  Demux4/3 -> [Icw1_rms]
  Demux4/2 -> [Ibw1_rms]
  Demux4/1 -> [Iaw1_rms]
  Demux5/1 -> [Va_rms]
  Demux5/2 -> [Vb_rms]
  Demux5/3 -> [Vc_rms]
  Demux2/1 -> Fcn/1
  Fcn/1 -> 50/51 Relays 06122015/2
  [Iabc_w1] -> 50/51 Relays 06122015/1
  50/51 Relays 06122015/1 -> Logical Operator/1
  [Ibw1_mag] -> Bus Creator1/3
  [Icw1_mag] -> Bus Creator1/5
  [Va_mag] -> Bus Creator1/7
  [Vb_mag] -> Bus Creator1/9
  [Vc_mag] -> Bus Creator1/11
  Gain10/1 -> Bus Creator1/13
  Gain6/1 -> Bus Creator1/14
  Gain7/1 -> Bus Creator1/15
  [Iaw1_rms] -> Bus Creator1/18
  [Icw1_rms] -> Bus Creator1/20
  [Ibw1_rms] -> Bus Creator1/19
  [Va_rms] -> Bus Creator1/21
  [Vb_rms] -> Bus Creator1/22
  [Vc_rms] -> Bus Creator1/23
  Logical Operator/1 -> Logic_trip/1
  Demux2/2 -> op_mode/1
  [Iaw1_phase] -> Bus Creator1/2
  [Ibw1_phase] -> Bus Creator1/4
  [Icw1_phase] -> Bus Creator1/6
  [Va_phase] -> Bus Creator1/8
  [Vb_phase] -> Bus Creator1/10
  [Vb_phase] -> Bus Creator1/12
  Constant/1 -> Bus Creator1/24
  Constant1/1 -> Bus Creator1/25
  [Vabc] -> Gain2/1
  Gain2/1 -> Demux/1
  [Iabc_w1] -> Gain3/1
  Gain3/1 -> ?
  Demux10/1 -> [Va_mag]
  Demux10/2 -> [Vb_mag]
  Demux10/3 -> [Vc_mag]
  Complex to Magnitude-Angle/1 -> Demux10/1
  [Vabc] -> Complex to Magnitude-Angle/1
  Complex to Magnitude-Angle1/1 -> Demux11/1
  [Iabc_w1] -> Complex to Magnitude-Angle1/1
  Demux11/1 -> [Iaw1_mag]
  Demux11/2 -> [Ibw1_mag]
  Demux11/3 -> [Icw1_mag]

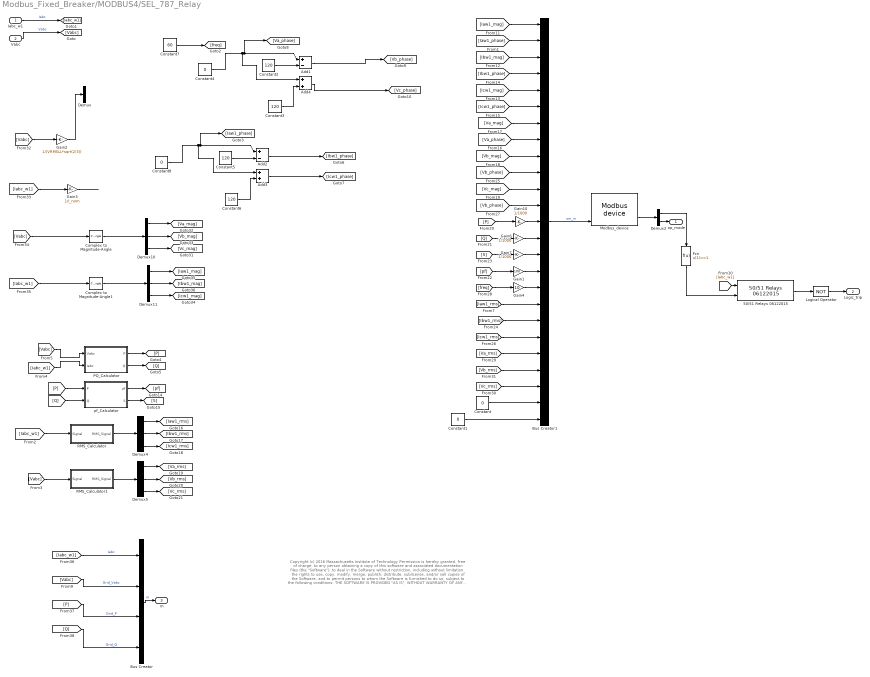
== system Modbus_Fixed_Breaker/MODBUS4/SEL_787_Relay ==
  note: Copyright (c) 2016 Massachusetts Institute of Technology
      | Permission is hereby granted, free of charge, to any person obtaining a copy of this software and associated documentation files (the "Software"), to deal
      | in the Software without restriction, including without limitation the rights to use, copy, modify, merge, publish, distribute, sublicense, and/or sell copies of the
      | Software, and to permit persons to whom the Software is furnished to do so, subject to the following conditions:
      |
      | THE SOFTWARE IS PROVIDED "AS IS", WITHOUT WARRANTY OF ANY KIND, EXPRESS OR IMPLIED, INCLUDING BUT NOT LIMITED TO THE
      | WARRANTIES OF MERCHANTABILITY, FITNESS FOR A PARTICULAR PURPOSE AND NONINFRINGEMENT. IN NO EVENT SHALL THE AUTHORS
      | OR COPYRIGHT HOLDERS BE LIABLE FOR ANY CLAIM, DAMAGES OR OTHER LIABILITY, WHETHER IN AN ACTION OF CONTRACT, TORT OR
      | OTHERWISE, ARISING FROM, OUT OF OR IN CONNECTION WITH THE SOFTWARE OR THE USE OR OTHER DEALINGS IN THE SOFTWARE
  Iabc_w1 : Inport
  Vabc : Inport  Port=2
  50/51 Relays 06122015 : breakers_1ph_3ph/50//51 Relays 06122015  TOC=TOC  IOC=IOC  Ts=Ts
  Add1 : Sum  Inputs=+-
  Add2 : Sum  Inputs=+-
  Add3 : Sum
  Add4 : Sum
  Bus Creator : BusCreator
  Bus Creator1 : BusCreator  Inputs=25
  Complex to Magnitude-Angle : ComplexToMagnitudeAngle  Output=Magnitude
  Complex to Magnitude-Angle1 : ComplexToMagnitudeAngle  Output=Magnitude
  Constant{,1,4,8} (4 alike) : Constant  Value=0
  Constant{2..3,5..6} (4 alike) : Constant  Value=120
  Constant7 : Constant  Value=60
  Demux{,4..5,10..11} (5 alike) : Demux  Outputs=3
  Demux2 : Demux  Outputs=2
  Fcn : Fcn  Expr=u(1)==1
  Gain1 : Gain  Gain=100
  Gain10 : Gain  Gain=1/1000
  Gain2 : Gain  Gain=1/(VRMSLL*sqrt(2/3))
  Gain3 : Gain  Gain=1/I_nom
  Gain4 : Gain  Gain=10
  Gain6 : Gain  Gain=1/1000
  Gain7 : Gain  Gain=1/1000
  Logical Operator : Logic  Operator=NOT  AllPortsSameDT=off  OutDataTypeStr=boolean
  Modbus_device : rtio_generic_modbus/Modbus device  conf_name=relay_slave_cfg1.opal  conf_name_mask=relay_slave_cfg4.xls  sample_time=Ts
  PQ_Calculator : Subsystem
  RMS_Calculator : Subsystem
  RMS_Calculator1 : Subsystem
  pf_Calculator : Subsystem
  op_mode : Outport
  Logic_trip : Outport  Port=2
  m : Outport  Port=3
  wires:
  Gain4/1 -> Bus Creator1/17
  Gain1/1 -> Bus Creator1/16
  [pf] -> Gain1/1
  [freq] -> Gain4/1
  Constant4/1 -> Add4/1, [Va_phase], Add1/1
  Add4/1 -> [Vc_phase]
  Add1/1 -> [Vb_phase]
  Constant3/1 -> Add4/2
  Constant2/1 -> Add1/2
  Constant8/1 -> Add3/1, [Iaw1_phase], Add2/1
  Add3/1 -> [Icw1_phase]
  Add2/1 -> [Ibw1_phase]
  Constant6/1 -> Add3/2
  Constant5/1 -> Add2/2
  Constant7/1 -> [freq]
  pf_Calculator/2(S) -> [S]
  Bus Creator1/1 -> Modbus_device/4  "sm_in"
  Modbus_device/2 -> Demux2/1
  [Q] -> Bus Creator/4  "Grid_Q"
  [P] -> Bus Creator/3  "Grid_P"
  [Vabc] -> Bus Creator/2  "Grid_Vabc"
  [Iabc_w1] -> Bus Creator/1  "Iabc"
  Bus Creator/1 -> m/1  "m"
  Iabc_w1/1 -> [Iabc_w1]  "Iabc"
  Vabc/1 -> [Vabc]  "Vabc"
  [Vabc] -> PQ_Calculator/1(Vabc)
  [Iabc_w1] -> PQ_Calculator/2(Iabc)
  [Iaw1_mag] -> Bus Creator1/1
  [P] -> Gain10/1
  [Q] -> Gain6/1
  [S] -> Gain7/1
  pf_Calculator/1(pf) -> [pf]
  [P] -> pf_Calculator/1(P)
  [Q] -> pf_Calculator/2(Q)
  PQ_Calculator/1(P) -> [P]
  PQ_Calculator/2(Q) -> [Q]
  [Iabc_w1] -> RMS_Calculator/1(Signal)
  [Vabc] -> RMS_Calculator1/1(Signal)
  RMS_Calculator/1(RMS_Signal) -> Demux4/1
  RMS_Calculator1/1(RMS_Signal) -> Demux5/1
  Demux4/3 -> [Icw1_rms]
  Demux4/2 -> [Ibw1_rms]
  Demux4/1 -> [Iaw1_rms]
  Demux5/1 -> [Va_rms]
  Demux5/2 -> [Vb_rms]
  Demux5/3 -> [Vc_rms]
  Demux2/1 -> Fcn/1
  Fcn/1 -> 50/51 Relays 06122015/2
  [Iabc_w1] -> 50/51 Relays 06122015/1
  50/51 Relays 06122015/1 -> Logical Operator/1
  [Ibw1_mag] -> Bus Creator1/3
  [Icw1_mag] -> Bus Creator1/5
  [Va_mag] -> Bus Creator1/7
  [Vb_mag] -> Bus Creator1/9
  [Vc_mag] -> Bus Creator1/11
  Gain10/1 -> Bus Creator1/13
  Gain6/1 -> Bus Creator1/14
  Gain7/1 -> Bus Creator1/15
  [Iaw1_rms] -> Bus Creator1/18
  [Icw1_rms] -> Bus Creator1/20
  [Ibw1_rms] -> Bus Creator1/19
  [Va_rms] -> Bus Creator1/21
  [Vb_rms] -> Bus Creator1/22
  [Vc_rms] -> Bus Creator1/23
  Logical Operator/1 -> Logic_trip/1
  Demux2/2 -> op_mode/1
  [Iaw1_phase] -> Bus Creator1/2
  [Ibw1_phase] -> Bus Creator1/4
  [Icw1_phase] -> Bus Creator1/6
  [Va_phase] -> Bus Creator1/8
  [Vb_phase] -> Bus Creator1/10
  [Vb_phase] -> Bus Creator1/12
  Constant/1 -> Bus Creator1/24
  Constant1/1 -> Bus Creator1/25
  [Vabc] -> Gain2/1
  Gain2/1 -> Demux/1
  [Iabc_w1] -> Gain3/1
  Gain3/1 -> ?
  Demux10/1 -> [Va_mag]
  Demux10/2 -> [Vb_mag]
  Demux10/3 -> [Vc_mag]
  Complex to Magnitude-Angle/1 -> Demux10/1
  [Vabc] -> Complex to Magnitude-Angle/1
  Complex to Magnitude-Angle1/1 -> Demux11/1
  [Iabc_w1] -> Complex to Magnitude-Angle1/1
  Demux11/1 -> [Iaw1_mag]
  Demux11/2 -> [Ibw1_mag]
  Demux11/3 -> [Icw1_mag]

== system Modbus_Fixed_Breaker/MODBUS1/SEL_787_Relay/PQ_Calculator ==
  Vabc : Inport
  Iabc : Inport  Port=2
  3-phase  Instantaneous  Active & Reactive Power : powerlib_extras/Measurements/3-phase  Instantaneous  Active & Reactive Power
  Demux : Demux  Outputs=2
  Discrete  Mean value2 : powerlib_extras/Discrete Measurements/Discrete  Mean value  Freq=60  Vinit=0  Ts=Ts
  P : Outport
  Q : Outport  Port=2
  wires:
  3-phase  Instantaneous  Active & Reactive Power/1 -> Discrete  Mean value2/1
  Discrete  Mean value2/1 -> Demux/1
  Vabc/1 -> 3-phase  Instantaneous  Active & Reactive Power/1
  Iabc/1 -> 3-phase  Instantaneous  Active & Reactive Power/2
  Demux/1 -> P/1  "P"
  Demux/2 -> Q/1  "Q"

== system Modbus_Fixed_Breaker/MODBUS1/SEL_787_Relay/RMS_Calculator ==
  Signal : Inport
  Discrete  Mean value6 : powerlib_extras/Discrete Measurements/Discrete  Mean value  Freq=60  Vinit=0  Ts=Ts
  Product3 : Product  RndMeth=Zero
  Signed Sqrt : Sqrt  SaturateOnIntegerOverflow=on
  RMS_Signal : Outport
  wires:
  Signal/1 -> Product3/1, Product3/2
  Product3/1 -> Discrete  Mean value6/1
  Discrete  Mean value6/1 -> Signed Sqrt/1
  Signed Sqrt/1 -> RMS_Signal/1

== system Modbus_Fixed_Breaker/MODBUS1/SEL_787_Relay/RMS_Calculator1 ==
  Signal : Inport
  Discrete  Mean value6 : powerlib_extras/Discrete Measurements/Discrete  Mean value  Freq=60  Vinit=0  Ts=Ts
  Product3 : Product  RndMeth=Zero
  Signed Sqrt : Sqrt  SaturateOnIntegerOverflow=on
  RMS_Signal : Outport
  wires:
  Signal/1 -> Product3/1, Product3/2
  Product3/1 -> Discrete  Mean value6/1
  Discrete  Mean value6/1 -> Signed Sqrt/1
  Signed Sqrt/1 -> RMS_Signal/1

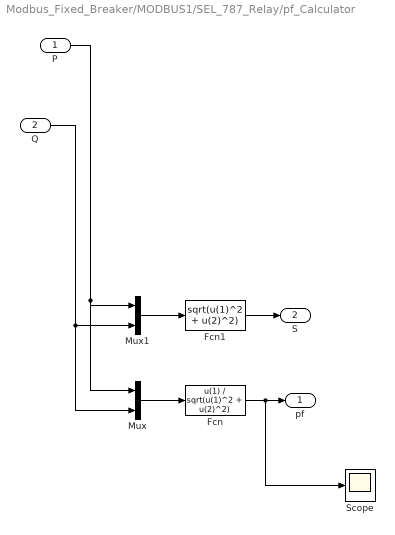
== system Modbus_Fixed_Breaker/MODBUS1/SEL_787_Relay/pf_Calculator ==
  P : Inport
  Q : Inport  Port=2
  Fcn : Fcn  Expr=u(1) / sqrt(u(1)^2 + u(2)^2)
  Fcn1 : Fcn  Expr=sqrt(u(1)^2 + u(2)^2)
  Mux : Mux  Inputs=2
  Mux1 : Mux  Inputs=2
  Scope : Scope
      settings: YMin=0.8475  YMax=0.875  SaveName=ScopeData2
  pf : Outport
  S : Outport  Port=2
  wires:
  Fcn1/1 -> S/1
  Mux1/1 -> Fcn1/1
  Fcn/1 -> Scope/1, pf/1
  Mux/1 -> Fcn/1
  P/1 -> Mux1/1, Mux/1
  Q/1 -> Mux1/2, Mux/2

== system Modbus_Fixed_Breaker/MODBUS2/SEL_787_Relay/PQ_Calculator ==
  Vabc : Inport
  Iabc : Inport  Port=2
  3-phase  Instantaneous  Active & Reactive Power : powerlib_extras/Measurements/3-phase  Instantaneous  Active & Reactive Power
  Demux : Demux  Outputs=2
  Discrete  Mean value2 : powerlib_extras/Discrete Measurements/Discrete  Mean value  Freq=60  Vinit=0  Ts=Ts
  P : Outport
  Q : Outport  Port=2
  wires:
  3-phase  Instantaneous  Active & Reactive Power/1 -> Discrete  Mean value2/1
  Discrete  Mean value2/1 -> Demux/1
  Vabc/1 -> 3-phase  Instantaneous  Active & Reactive Power/1
  Iabc/1 -> 3-phase  Instantaneous  Active & Reactive Power/2
  Demux/1 -> P/1  "P"
  Demux/2 -> Q/1  "Q"

== system Modbus_Fixed_Breaker/MODBUS2/SEL_787_Relay/RMS_Calculator ==
  Signal : Inport
  Discrete  Mean value6 : powerlib_extras/Discrete Measurements/Discrete  Mean value  Freq=60  Vinit=0  Ts=Ts
  Product3 : Product  RndMeth=Zero
  Signed Sqrt : Sqrt  SaturateOnIntegerOverflow=on
  RMS_Signal : Outport
  wires:
  Signal/1 -> Product3/1, Product3/2
  Product3/1 -> Discrete  Mean value6/1
  Discrete  Mean value6/1 -> Signed Sqrt/1
  Signed Sqrt/1 -> RMS_Signal/1

== system Modbus_Fixed_Breaker/MODBUS2/SEL_787_Relay/RMS_Calculator1 ==
  Signal : Inport
  Discrete  Mean value6 : powerlib_extras/Discrete Measurements/Discrete  Mean value  Freq=60  Vinit=0  Ts=Ts
  Product3 : Product  RndMeth=Zero
  Signed Sqrt : Sqrt  SaturateOnIntegerOverflow=on
  RMS_Signal : Outport
  wires:
  Signal/1 -> Product3/1, Product3/2
  Product3/1 -> Discrete  Mean value6/1
  Discrete  Mean value6/1 -> Signed Sqrt/1
  Signed Sqrt/1 -> RMS_Signal/1

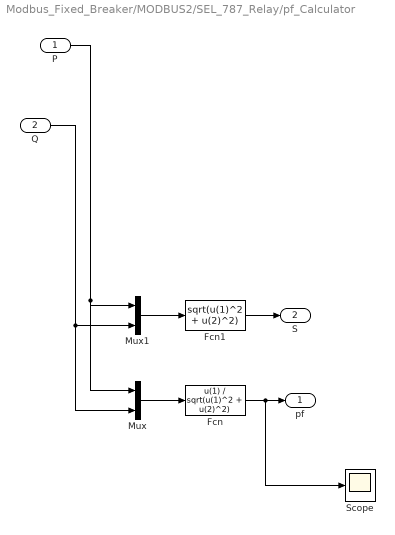
== system Modbus_Fixed_Breaker/MODBUS2/SEL_787_Relay/pf_Calculator ==
  P : Inport
  Q : Inport  Port=2
  Fcn : Fcn  Expr=u(1) / sqrt(u(1)^2 + u(2)^2)
  Fcn1 : Fcn  Expr=sqrt(u(1)^2 + u(2)^2)
  Mux : Mux  Inputs=2
  Mux1 : Mux  Inputs=2
  Scope : Scope
      settings: YMin=0.8475  YMax=0.875  SaveName=ScopeData2
  pf : Outport
  S : Outport  Port=2
  wires:
  Fcn1/1 -> S/1
  Mux1/1 -> Fcn1/1
  Fcn/1 -> Scope/1, pf/1
  Mux/1 -> Fcn/1
  P/1 -> Mux1/1, Mux/1
  Q/1 -> Mux1/2, Mux/2

== system Modbus_Fixed_Breaker/MODBUS3/SEL_787_Relay/PQ_Calculator ==
  Vabc : Inport
  Iabc : Inport  Port=2
  3-phase  Instantaneous  Active & Reactive Power : powerlib_extras/Measurements/3-phase  Instantaneous  Active & Reactive Power
  Demux : Demux  Outputs=2
  Discrete  Mean value2 : powerlib_extras/Discrete Measurements/Discrete  Mean value  Freq=60  Vinit=0  Ts=Ts
  P : Outport
  Q : Outport  Port=2
  wires:
  3-phase  Instantaneous  Active & Reactive Power/1 -> Discrete  Mean value2/1
  Discrete  Mean value2/1 -> Demux/1
  Vabc/1 -> 3-phase  Instantaneous  Active & Reactive Power/1
  Iabc/1 -> 3-phase  Instantaneous  Active & Reactive Power/2
  Demux/1 -> P/1  "P"
  Demux/2 -> Q/1  "Q"

== system Modbus_Fixed_Breaker/MODBUS3/SEL_787_Relay/RMS_Calculator ==
  Signal : Inport
  Discrete  Mean value6 : powerlib_extras/Discrete Measurements/Discrete  Mean value  Freq=60  Vinit=0  Ts=Ts
  Product3 : Product  RndMeth=Zero
  Signed Sqrt : Sqrt  SaturateOnIntegerOverflow=on
  RMS_Signal : Outport
  wires:
  Signal/1 -> Product3/1, Product3/2
  Product3/1 -> Discrete  Mean value6/1
  Discrete  Mean value6/1 -> Signed Sqrt/1
  Signed Sqrt/1 -> RMS_Signal/1

== system Modbus_Fixed_Breaker/MODBUS3/SEL_787_Relay/RMS_Calculator1 ==
  Signal : Inport
  Discrete  Mean value6 : powerlib_extras/Discrete Measurements/Discrete  Mean value  Freq=60  Vinit=0  Ts=Ts
  Product3 : Product  RndMeth=Zero
  Signed Sqrt : Sqrt  SaturateOnIntegerOverflow=on
  RMS_Signal : Outport
  wires:
  Signal/1 -> Product3/1, Product3/2
  Product3/1 -> Discrete  Mean value6/1
  Discrete  Mean value6/1 -> Signed Sqrt/1
  Signed Sqrt/1 -> RMS_Signal/1

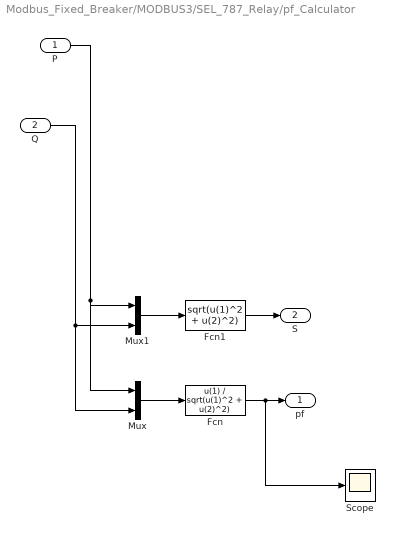
== system Modbus_Fixed_Breaker/MODBUS3/SEL_787_Relay/pf_Calculator ==
  P : Inport
  Q : Inport  Port=2
  Fcn : Fcn  Expr=u(1) / sqrt(u(1)^2 + u(2)^2)
  Fcn1 : Fcn  Expr=sqrt(u(1)^2 + u(2)^2)
  Mux : Mux  Inputs=2
  Mux1 : Mux  Inputs=2
  Scope : Scope
      settings: YMin=0.8475  YMax=0.875  SaveName=ScopeData2
  pf : Outport
  S : Outport  Port=2
  wires:
  Fcn1/1 -> S/1
  Mux1/1 -> Fcn1/1
  Fcn/1 -> Scope/1, pf/1
  Mux/1 -> Fcn/1
  P/1 -> Mux1/1, Mux/1
  Q/1 -> Mux1/2, Mux/2

== system Modbus_Fixed_Breaker/MODBUS4/SEL_787_Relay/PQ_Calculator ==
  Vabc : Inport
  Iabc : Inport  Port=2
  3-phase  Instantaneous  Active & Reactive Power : powerlib_extras/Measurements/3-phase  Instantaneous  Active & Reactive Power
  Demux : Demux  Outputs=2
  Discrete  Mean value2 : powerlib_extras/Discrete Measurements/Discrete  Mean value  Freq=60  Vinit=0  Ts=Ts
  P : Outport
  Q : Outport  Port=2
  wires:
  3-phase  Instantaneous  Active & Reactive Power/1 -> Discrete  Mean value2/1
  Discrete  Mean value2/1 -> Demux/1
  Vabc/1 -> 3-phase  Instantaneous  Active & Reactive Power/1
  Iabc/1 -> 3-phase  Instantaneous  Active & Reactive Power/2
  Demux/1 -> P/1  "P"
  Demux/2 -> Q/1  "Q"

== system Modbus_Fixed_Breaker/MODBUS4/SEL_787_Relay/RMS_Calculator ==
  Signal : Inport
  Discrete  Mean value6 : powerlib_extras/Discrete Measurements/Discrete  Mean value  Freq=60  Vinit=0  Ts=Ts
  Product3 : Product  RndMeth=Zero
  Signed Sqrt : Sqrt  SaturateOnIntegerOverflow=on
  RMS_Signal : Outport
  wires:
  Signal/1 -> Product3/1, Product3/2
  Product3/1 -> Discrete  Mean value6/1
  Discrete  Mean value6/1 -> Signed Sqrt/1
  Signed Sqrt/1 -> RMS_Signal/1

== system Modbus_Fixed_Breaker/MODBUS4/SEL_787_Relay/RMS_Calculator1 ==
  Signal : Inport
  Discrete  Mean value6 : powerlib_extras/Discrete Measurements/Discrete  Mean value  Freq=60  Vinit=0  Ts=Ts
  Product3 : Product  RndMeth=Zero
  Signed Sqrt : Sqrt  SaturateOnIntegerOverflow=on
  RMS_Signal : Outport
  wires:
  Signal/1 -> Product3/1, Product3/2
  Product3/1 -> Discrete  Mean value6/1
  Discrete  Mean value6/1 -> Signed Sqrt/1
  Signed Sqrt/1 -> RMS_Signal/1

== system Modbus_Fixed_Breaker/MODBUS4/SEL_787_Relay/pf_Calculator ==
  P : Inport
  Q : Inport  Port=2
  Fcn : Fcn  Expr=u(1) / sqrt(u(1)^2 + u(2)^2)
  Fcn1 : Fcn  Expr=sqrt(u(1)^2 + u(2)^2)
  Mux : Mux  Inputs=2
  Mux1 : Mux  Inputs=2
  Scope : Scope
      settings: YMin=0.8475  YMax=0.875  SaveName=ScopeData2
  pf : Outport
  S : Outport  Port=2
  wires:
  Fcn1/1 -> S/1
  Mux1/1 -> Fcn1/1
  Fcn/1 -> Scope/1, pf/1
  Mux/1 -> Fcn/1
  P/1 -> Mux1/1, Mux/1
  Q/1 -> Mux1/2, Mux/2
